simulink model "test_dac"  (Simulink 7.6)
settings: Solver=FixedStepDiscrete  StartTime=0.0  StopTime=800  FixedStep=1  RelTol=1e-3
libraries: simulink x23
settings Model: Creator=jordan  LastModifiedBy=jordan
settings DataIOCC: LimitDataPoints=off  SaveOutput=off  SignalLogging=off  DSMLogging=off  SaveTime=off
settings OptimizationCC: BlockReduction=off  ConditionallyExecuteInputs=off  InlineParams=on

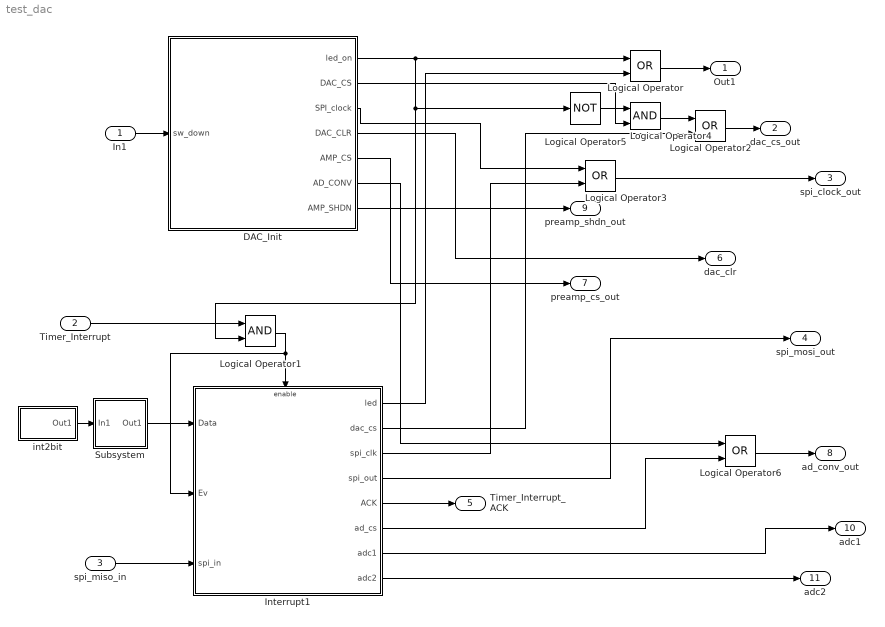
== system test_dac ==
  In1 : Inport  OutDataTypeStr=boolean
  Timer_Interrupt : Inport  Port=2  OutDataTypeStr=boolean
  spi_miso_in : Inport  Port=3  OutDataTypeStr=boolean
  DAC_Init : Stateflow chart  TreatAsAtomicUnit=on
  Interrupt1 : Subsystem
  Logical Operator{,2..3,6} (4 alike) : Logic  Operator=OR  AllPortsSameDT=off  OutDataTypeStr=boolean
  Logical Operator1 : Logic  AllPortsSameDT=off  OutDataTypeStr=boolean
  Logical Operator4 : Logic  AllPortsSameDT=off  OutDataTypeStr=boolean
  Logical Operator5 : Logic  Operator=NOT  AllPortsSameDT=off  OutDataTypeStr=boolean
  Subsystem : Subsystem
  int2bit : Subsystem
  Out1 : Outport
  dac_cs_out : Outport  Port=2
  spi_clock_out : Outport  Port=3
  spi_mosi_out : Outport  Port=4
  Timer_Interrupt_ACK : Outport  Port=5
  dac_clr : Outport  Port=6
  preamp_cs_out : Outport  Port=7
  ad_conv_out : Outport  Port=8
  preamp_shdn_out : Outport  Port=9
  adc1 : Outport  Port=10
  adc2 : Outport  Port=11
  wires:
  In1/1 -> DAC_Init/1(sw_down)
  Timer_Interrupt/1 -> Logical Operator1/1
  Interrupt1/5(ACK) -> Timer_Interrupt_ACK/1
  Subsystem/1(Out1) -> Interrupt1/1(Data)
  DAC_Init/1(led_on) -> Logical Operator/1, Logical Operator1/2, Logical Operator5/1
  Logical Operator1/1 -> Interrupt1/Enable, Interrupt1/2(Ev)
  Interrupt1/1(led) -> Logical Operator/2
  Logical Operator/1 -> Out1/1
  Logical Operator2/1 -> dac_cs_out/1
  DAC_Init/2(DAC_CS) -> Logical Operator4/2
  Interrupt1/2(dac_cs) -> Logical Operator2/2
  Logical Operator3/1 -> spi_clock_out/1
  DAC_Init/3(SPI_clock) -> Logical Operator3/1
  Interrupt1/3(spi_clk) -> Logical Operator3/2
  Interrupt1/4(spi_out) -> spi_mosi_out/1
  DAC_Init/4(DAC_CLR) -> dac_clr/1
  Logical Operator4/1 -> Logical Operator2/1
  Logical Operator5/1 -> Logical Operator4/1
  int2bit/1(Out1) -> Subsystem/1(In1)
  DAC_Init/5(AMP_CS) -> preamp_cs_out/1
  DAC_Init/6(AD_CONV) -> Logical Operator6/1
  spi_miso_in/1 -> Interrupt1/3(spi_in)
  DAC_Init/7(AMP_SHDN) -> preamp_shdn_out/1
  Logical Operator6/1 -> ad_conv_out/1
  Interrupt1/6(ad_cs) -> Logical Operator6/2
  Interrupt1/7(adc1) -> adc1/1
  Interrupt1/8(adc2) -> adc2/1

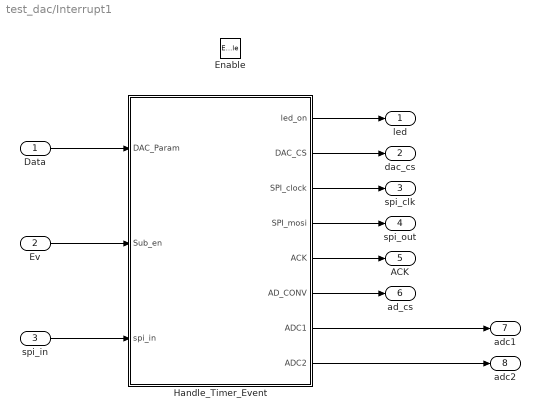
== system test_dac/Interrupt1 ==
  Data : Inport  OutDataTypeStr=boolean
  Ev : Inport  Port=2  OutDataTypeStr=boolean
  spi_in : Inport  Port=3  OutDataTypeStr=boolean
  Enable : EnablePort
  Handle_Timer_Event : Stateflow chart  TreatAsAtomicUnit=on
  led : Outport  InitialOutput=0
  dac_cs : Outport  Port=2  InitialOutput=0
  spi_clk : Outport  Port=3  InitialOutput=0
  spi_out : Outport  Port=4  InitialOutput=0
  ACK : Outport  Port=5  InitialOutput=0
  ad_cs : Outport  Port=6  InitialOutput=0
  adc1 : Outport  Port=7  InitialOutput=0
  adc2 : Outport  Port=8  InitialOutput=0
  wires:
  Handle_Timer_Event/1(led_on) -> led/1
  Handle_Timer_Event/2(DAC_CS) -> dac_cs/1
  Handle_Timer_Event/3(SPI_clock) -> spi_clk/1
  Handle_Timer_Event/4(SPI_mosi) -> spi_out/1
  Data/1 -> Handle_Timer_Event/1(DAC_Param)
  Handle_Timer_Event/5(ACK) -> ACK/1
  Ev/1 -> Handle_Timer_Event/2(Sub_en)
  spi_in/1 -> Handle_Timer_Event/3(spi_in)
  Handle_Timer_Event/6(AD_CONV) -> ad_cs/1
  Handle_Timer_Event/8(ADC2) -> adc2/1
  Handle_Timer_Event/7(ADC1) -> adc1/1

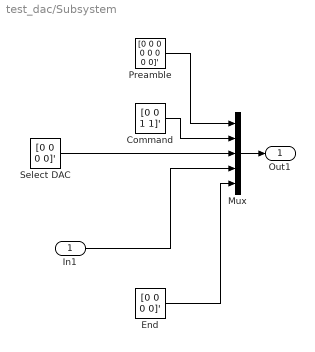
== system test_dac/Subsystem ==
  In1 : Inport  OutDataTypeStr=boolean
  Command : Constant  Value=[0 0 1 1]'  OutDataTypeStr=boolean
  End : Constant  Value=[0 0 0 0]'  OutDataTypeStr=boolean
  Mux : Mux  Inputs=5
  Preamble : Constant  Value=[0 0 0 0 0 0 0 0]'  OutDataTypeStr=boolean
  Select DAC : Constant  Value=[0 0 0 0]'  OutDataTypeStr=boolean
  Out1 : Outport
  wires:
  Preamble/1 -> Mux/1
  Command/1 -> Mux/2
  Select DAC/1 -> Mux/3
  In1/1 -> Mux/4
  End/1 -> Mux/5
  Mux/1 -> Out1/1

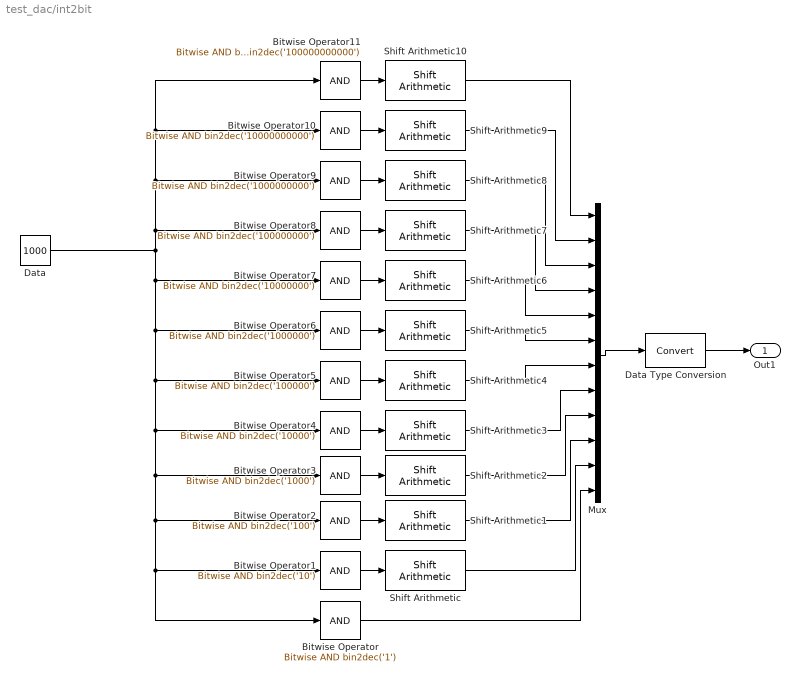
== system test_dac/int2bit ==
  Bitwise Operator : simulink/Logic and Bit Operations/Bitwise Operator  logicop=AND  UseBitMask=on  BitMask=bin2dec('1')  BitMaskRealWorld=Stored Integer
  Bitwise Operator1 : simulink/Logic and Bit Operations/Bitwise Operator  logicop=AND  UseBitMask=on  BitMask=bin2dec('10')  BitMaskRealWorld=Stored Integer
  Bitwise Operator10 : simulink/Logic and Bit Operations/Bitwise Operator  logicop=AND  UseBitMask=on  BitMask=bin2dec('10000000000')  BitMaskRealWorld=Stored Integer
  Bitwise Operator11 : simulink/Logic and Bit Operations/Bitwise Operator  logicop=AND  UseBitMask=on  BitMask=bin2dec('100000000000')  BitMaskRealWorld=Stored Integer
  Bitwise Operator2 : simulink/Logic and Bit Operations/Bitwise Operator  logicop=AND  UseBitMask=on  BitMask=bin2dec('100')  BitMaskRealWorld=Stored Integer
  Bitwise Operator3 : simulink/Logic and Bit Operations/Bitwise Operator  logicop=AND  UseBitMask=on  BitMask=bin2dec('1000')  BitMaskRealWorld=Stored Integer
  Bitwise Operator4 : simulink/Logic and Bit Operations/Bitwise Operator  logicop=AND  UseBitMask=on  BitMask=bin2dec('10000')  BitMaskRealWorld=Stored Integer
  Bitwise Operator5 : simulink/Logic and Bit Operations/Bitwise Operator  logicop=AND  UseBitMask=on  BitMask=bin2dec('100000')  BitMaskRealWorld=Stored Integer
  Bitwise Operator6 : simulink/Logic and Bit Operations/Bitwise Operator  logicop=AND  UseBitMask=on  BitMask=bin2dec('1000000')  BitMaskRealWorld=Stored Integer
  Bitwise Operator7 : simulink/Logic and Bit Operations/Bitwise Operator  logicop=AND  UseBitMask=on  BitMask=bin2dec('10000000')  BitMaskRealWorld=Stored Integer
  Bitwise Operator8 : simulink/Logic and Bit Operations/Bitwise Operator  logicop=AND  UseBitMask=on  BitMask=bin2dec('100000000')  BitMaskRealWorld=Stored Integer
  Bitwise Operator9 : simulink/Logic and Bit Operations/Bitwise Operator  logicop=AND  UseBitMask=on  BitMask=bin2dec('1000000000')  BitMaskRealWorld=Stored Integer
  Data : Constant  Value=1000  OutDataTypeStr=fixdt(0,12,0)
  Data Type Conversion : DataTypeConversion
  Mux : Mux  Inputs=12
  Shift Arithmetic : simulink/Logic and Bit Operations/Shift Arithmetic  SystemSampleTime=-1  nBitShiftRight=1  nBinPtShiftRight=0
  Shift Arithmetic1 : simulink/Logic and Bit Operations/Shift Arithmetic  SystemSampleTime=-1  nBitShiftRight=2  nBinPtShiftRight=0
  Shift Arithmetic10 : simulink/Logic and Bit Operations/Shift Arithmetic  SystemSampleTime=-1  nBitShiftRight=11  nBinPtShiftRight=0
  Shift Arithmetic2 : simulink/Logic and Bit Operations/Shift Arithmetic  SystemSampleTime=-1  nBitShiftRight=3  nBinPtShiftRight=0
  Shift Arithmetic3 : simulink/Logic and Bit Operations/Shift Arithmetic  SystemSampleTime=-1  nBitShiftRight=4  nBinPtShiftRight=0
  Shift Arithmetic4 : simulink/Logic and Bit Operations/Shift Arithmetic  SystemSampleTime=-1  nBitShiftRight=5  nBinPtShiftRight=0
  Shift Arithmetic5 : simulink/Logic and Bit Operations/Shift Arithmetic  SystemSampleTime=-1  nBitShiftRight=6  nBinPtShiftRight=0
  Shift Arithmetic6 : simulink/Logic and Bit Operations/Shift Arithmetic  SystemSampleTime=-1  nBitShiftRight=7  nBinPtShiftRight=0
  Shift Arithmetic7 : simulink/Logic and Bit Operations/Shift Arithmetic  SystemSampleTime=-1  nBitShiftRight=8  nBinPtShiftRight=0
  Shift Arithmetic8 : simulink/Logic and Bit Operations/Shift Arithmetic  SystemSampleTime=-1  nBitShiftRight=9  nBinPtShiftRight=0
  Shift Arithmetic9 : simulink/Logic and Bit Operations/Shift Arithmetic  SystemSampleTime=-1  nBitShiftRight=10  nBinPtShiftRight=0
  Out1 : Outport  InitialOutput=0
  wires:
  Data/1 -> Bitwise Operator11/1, Bitwise Operator10/1, Bitwise Operator9/1, Bitwise Operator8/1, Bitwise Operator7/1, Bitwise Operator6/1, Bitwise Operator5/1, Bitwise Operator4/1, Bitwise Operator3/1, Bitwise Operator2/1, Bitwise Operator/1, Bitwise Operator1/1
  Bitwise Operator1/1 -> Shift Arithmetic/1
  Bitwise Operator2/1 -> Shift Arithmetic1/1
  Bitwise Operator3/1 -> Shift Arithmetic2/1
  Bitwise Operator4/1 -> Shift Arithmetic3/1
  Bitwise Operator5/1 -> Shift Arithmetic4/1
  Bitwise Operator6/1 -> Shift Arithmetic5/1
  Bitwise Operator7/1 -> Shift Arithmetic6/1
  Bitwise Operator8/1 -> Shift Arithmetic7/1
  Bitwise Operator9/1 -> Shift Arithmetic8/1
  Bitwise Operator10/1 -> Shift Arithmetic9/1
  Bitwise Operator11/1 -> Shift Arithmetic10/1
  Bitwise Operator/1 -> Mux/12
  Shift Arithmetic/1 -> Mux/11
  Shift Arithmetic1/1 -> Mux/10
  Shift Arithmetic2/1 -> Mux/9
  Shift Arithmetic3/1 -> Mux/8
  Shift Arithmetic4/1 -> Mux/7
  Shift Arithmetic5/1 -> Mux/6
  Shift Arithmetic6/1 -> Mux/5
  Shift Arithmetic7/1 -> Mux/4
  Shift Arithmetic8/1 -> Mux/3
  Shift Arithmetic9/1 -> Mux/2
  Shift Arithmetic10/1 -> Mux/1
  Mux/1 -> Data Type Conversion/1
  Data Type Conversion/1 -> Out1/1

== stateflow chart Interrupt1/Handle_Timer_Event ==
  settings: executeAtInitialization=1
  state Led_is_On
  state Led_is_Off
  state End_of_Interrupt
  state Wait1
  state Wait3
  state Wait7
  state Wait8
  state AD_Start
  state Wait9
  state Wait10
  state Wait11
  state Wait12
  (default) -> Led_is_Off
  Led_is_Off -> Led_is_On : {DAC_CS=0;
      | ind1=0;
      | ACK=0;}
  Wait1 -> Wait7 : {SPI_clock=1;}
  Wait3 -> (junction 15)
  Wait7 -> Wait3 : {ind1++;
      | led_on=0;
      | SPI_clock=0;}
  (junction 15) -> (junction 16) [order 1] : [ind1<32]
  (junction 16) -> Wait1 : {SPI_mosi=DAC_Param[ind1];}
  Led_is_On -> (junction 15)
  (junction 15) -> AD_Start [order 2] : {DAC_CS=1;}
  End_of_Interrupt -> Wait8 : {ACK=0;}
  Wait8 -> Led_is_Off : [Sub_en==1]
  AD_Start -> Wait9 : {AD_CONV=1;}
  Wait9 -> Wait10 : {AD_CONV=0;
      | adc_data1=0;
      | adc_data2=0;
      | ind1=0;}
  Wait10 -> Wait11 : {SPI_clock=1;}
  Wait11 -> Wait12 : {SPI_clock=0;
      | ind1++;}
  Wait12 -> (junction 17) [order 1] : [ind1<34]
  (junction 17) -> (junction 18) [order 2] : [(ind1>1)&&(ind1<16)]{
      | adc_data1=adc_data1<<1;
      | adc_data1=adc_data1|spi_in;}
  (junction 17) -> (junction 18) [order 3]
  (junction 18) -> Wait10
  (junction 17) -> (junction 18) [order 1] : [(ind1>17)&&(ind1<32)]{
      | adc_data2=adc_data2<<1;
      | adc_data2=adc_data2|spi_in;}
  Wait12 -> End_of_Interrupt [order 2] : {ACK=1;
      | ADC1=adc_data1;
      | ADC2=adc_data2;}
  data: led_on output boolean; DAC_CS output boolean =1; SPI_clock output boolean =0; SPI_mosi output boolean; DAC_Param input boolean size=32; ind1 local uint8; ACK output boolean =0; Sub_en input boolean; adc_data1 local uint16; adc_data2 local uint16; spi_in input boolean; AD_CONV output boolean; ADC1 output uint16; ADC2 output uint16

== stateflow chart DAC_Init ==
  settings: executeAtInitialization=1
  state DAC_init
  state Led_is_Off
  state Wait6
  state Wait3
  state Wait7
  state Wait8
  state Wait9
  state AMP_Init
  (default) -> Led_is_Off
  Led_is_Off -> DAC_init : {SPI_clock=0;
      | DAC_CS=1;
      | DAC_CLR=1;
      | AMP_CS=1; AMP_SHDN=1;
      | AD_CONV=0;
      | ind1=0;}
  Wait6 -> AMP_Init : {DAC_CLR=1;
      | led_on=1;}
  Wait7 -> (junction 64)
  (junction 65) -> Wait3 : {ind1++;}
  (junction 64) -> (junction 65) [order 1] : [ind1<255]
  (junction 64) -> Wait6 [order 2] : {DAC_CLR=0;}
  DAC_init -> (junction 64)
  Wait3 -> Wait9
  Wait9 -> Wait8
  Wait8 -> Wait7
  data: sw_down input boolean =0; led_on output boolean; DAC_CS output boolean =1; SPI_clock output boolean =0; DAC_CLR output boolean =1; ind1 local uint8; AMP_CS output boolean; AD_CONV output boolean; AMP_SHDN output boolean
